simulink model "pa_measure"  (R2014a)
settings: Solver=FixedStepDiscrete  SolverMode=SingleTasking  StartTime=0.0  StopTime=inf  RelTol=1e-3
PreLoadFcn:
  | Fs = 10e6;
  | filter_num=[ .25]*exp(j*pi/4);     % phase offset
  | filter_den=[1 -.75*(1+j)/sqrt(2)]; % complex denominator
StartFcn:
  | tic
StopFcn:
  | trun=toc
undefined symbols (not defined in the file or in its folder): dfilt, fdesignblkfcn, gcbh
libraries: dsparch4 x2, commchan3 x1, simulink x1, commrflib2 x1
settings Model: Creator=Dick  LastModifiedBy=kschutz
settings DataIOCC: SaveOutput=off  SaveTime=off
settings OptimizationCC: BlockReduction=off  ConditionallyExecuteInputs=off  InlineParams=on  ExpressionDepthLimit=2147483647  SimCompilerOptimization=On
settings DebuggingCC: AlgebraicLoopMsg=error  UnderspecifiedInitializationDetection=Classic  InheritedTsInSrcMsg=none  MultiTaskRateTransMsg=warning  ParameterPrecisionLossMsg=none  FcnCallInpInsideContextMsg=EnableAllAsWarning  UnconnectedInputMsg=none  UnconnectedOutputMsg=none  StateNameClashWarn=warning
settings HardwareCC: ProdHWDeviceType=ASIC/FPGA->ASIC/FPGA  ProdEqTarget=off
settings SFSimCC: SimCtrlC=off
settings GRTTargetCC: CombineOutputUpdateFcns=off  GRTInterface=on

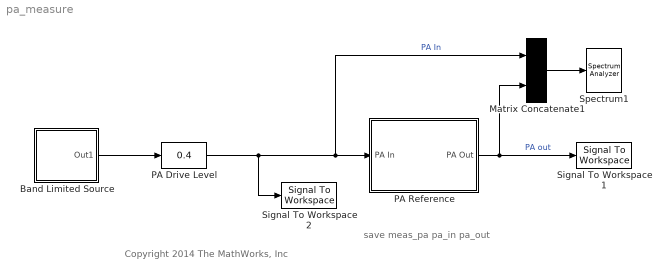
== system pa_measure ==
  note: Copyright 2014 The MathWorks, Inc
  note: save meas_pa pa_in pa_out
  " Spectrum1" : SpectrumAnalyzer
  Band Limited Source : Subsystem
  Matrix Concatenate1 : Concatenate  Mode=Multidimensional array  ConcatenateDimension=2
  PA Drive Level : simulink/Math Operations/Slider Gain  low=0  gain=0.4  high=1
  PA Reference : Subsystem
  Signal To Workspace 1 : SignalToWorkspace  VariableName=pa_out
      settings: CopyFcn=dspblkcopystw(gcbh);
  Signal To Workspace 2 : SignalToWorkspace  VariableName=pa_in
      settings: CopyFcn=dspblkcopystw(gcbh);
  wires:
  Band Limited Source/1(Out1) -> PA Drive Level/1
  PA Drive Level/1 -> PA Reference/1(PA In), Matrix Concatenate1/1, Signal To Workspace 2/1  "PA In"
  PA Reference/1(PA Out) -> Signal To Workspace 1/1, Matrix Concatenate1/2  "PA out"
  Matrix Concatenate1/1 -> " Spectrum1"/1

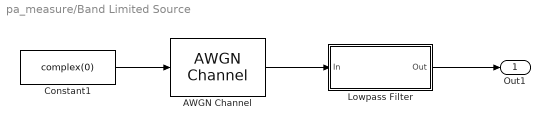
== system pa_measure/Band Limited Source ==
  AWGN Channel : commchan3/AWGN Channel  InputProcessing=Columns as channels (frame based)  seed=67  noiseMode=Variance from mask  EbNodB=10  EsNodB=10  SNRdB=10  bitsPerSym=1  Ps=1  Tsym=1  variance=1
  Constant1 : Constant  Value=complex(0)  VectorParams1D=off  SampleTime=1/Fs
  Lowpass Filter : Subsystem  DialogController=fdesignblkfcn  InitFcn=fdesignblkfcn(gcbh, {'InitFcn'});  mask(Lowpass Filter){}
      mask help: Design a lowpass filter
      settings: CopyFcn=fdesignblkfcn(gcbh, {'CopyFcn'});
      mask Help: helpview(mapfilelocation('dsp'), 'dsplowpassfilter');
      mask Display: disp('Lowpass')
  Out1 : Outport
  wires:
  Constant1/1 -> AWGN Channel/1
  Lowpass Filter/1(Out) -> Out1/1
  AWGN Channel/1 -> Lowpass Filter/1(In)

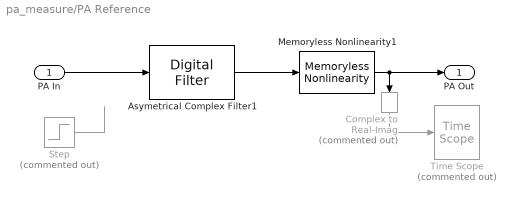
== system pa_measure/PA Reference ==
  PA In : Inport
  Asymetrical Complex Filter1 : dsparch4/Digital Filter  TypePopup=IIR (poles & zeros)  IIRFiltStruct=Direct form II transposed  AllPoleFiltStruct=Direct form  FIRFiltStruct=Direct form  CoeffSource=Specify via dialog  NumCoeffs="[0 filter_num]  % additional unit delay"  DenCoeffs=filter_den  BiQuadCoeffs=[1 0.3 0.4 1 0.1 0.2]  LatticeCoeffs=[0.2 0.4]  denIgnore=on  FiltPerSampPopup=One filter per frame  IC=0  ICnum=0  ICden=0  roundingMode=Floor  overflowMode=off  ScaleValues=1  scaleValueFracLength=14  stageInFracLength=15  stageOutFracLength=15  FilterSource=Specify via dialog  dfiltObjectName=dfilt.dffir([1 2 1])  InputProcessing=Columns as channels (frame based)
  Complex to Real-Imag : ComplexToRealImag  Commented=on  Output=Real
  Memoryless Nonlinearity1 : commrflib2/Memoryless Nonlinearity  model_select=Saleh model  linGaindB=0  GindB=-10  iip3=40  am2pm=10  LPwrLimAMPM=10  UPwrLimAMPM=inf  amam=[2.1587 1.1517]  ampm=[4.0033 9.1040]  x=[8.1081 1.5413 6.5202 -0.0718]  y=[4.6645 2.0965 10.88 -0.003]  p=0.5  GoutdB=31  vsat=1
  Step : Step  Commented=on  Time=1/Fs  SampleTime=1/Fs
  Time Scope : TimeScope  Commented=on  DefaultConfigurationName=spbscopes.TimeScopeBlockCfg
  PA Out : Outport
  wires:
  Asymetrical Complex Filter1/1 -> Memoryless Nonlinearity1/1
  Memoryless Nonlinearity1/1 -> PA Out/1, Complex to Real-Imag/1
  Complex to Real-Imag/1 -> Time Scope/1
  PA In/1 -> Asymetrical Complex Filter1/1
  Step/1 -> ?

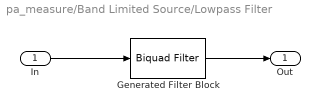
== system pa_measure/Band Limited Source/Lowpass Filter ==
  In : Inport
  Generated Filter Block : dsparch4/Biquad Filter  Tag=BlockMethodSubSystem  IIRFiltStruct=Direct form II  CoeffSource=Specify via dialog  BiQuadCoeffs=[0.59857121639186728 0.13537231817349551 0.59857121639186728 1 -0.91924875050540011 0.79125023824409946;0.071302617967318405 0.071302617967318405 0 1 -0.72689076105008177 0;1.9999999999999993 -0.61982790413552502 2 1 -0.61172653799164256 0.97438669274901857;0.10076583159845166 0.11489786555202355 0.10076583159845166 1 -1.2555266743020157 0.62505447110737744;2 -0.34405123549902639 1.9999999999999996 1 -0.69965198413855145 0.90732338685750258]  a0Flag=Warning  IC=0  ICnum=0  ICden=0  InputProcessing=Columns as channels (frame based)  denAccumFracLength=30  denProdOutputFracLength=30  secondMemoryFracLength=15  roundingMode=Floor  overflowMode=off  ScaleValues=[0.17872347192286847;1;1;1;1;1.090516053438453]  optimizeScaleValues=off  ScaleValueMode=Specify via input port (g)  scaleValueFracLength=14  FilterSource=Specify via dialog  dfiltObjectName=dfilt.df2tsos([1 0.3 0.4],[1 0.1 0.2])
  Out : Outport
  wires:
  In/1 -> Generated Filter Block/1
  Generated Filter Block/1 -> Out/1
